simulink model "model"  (R2020a)
settings: Solver=FixedStepAuto  StartTime=0.0  StopTime=20  FixedStep=0.0001  RelTol=1e-3
values from neighbouring files (symbols this model uses):
  alp = Iz1 + (r1^2)*m1 + (l1^2)*m2 + (l1^2)*m3 + (l1^2)*m4    (= 1.69)    [Parameters.m]
  beta = Iz1 + Iz2 + Iz3 + Iz4 + (l2^2)*m3+ (l2^2)*m4 +m2*(r2^2)    (= 1.803225)    [Parameters.m]
  Ct_States1 = [Ct_States1;[x1, x2, x3, x4]]    [Parameters.m]
  Ct_timeS = [Ct_timeS;t]    [Parameters.m]
  d1 = 1.5    [Parameters.m]
  del = Iz3 + Iz4    (= 0.0201)    [Parameters.m]
  g = 9.81    [Parameters.m]
  gam = l1*l2*m3 + l1*l2*m4 + l1*m2*r2    (= 1.15)    [Parameters.m]
  k1 = 600    [Parameters.m]
  k2 = 100    [Parameters.m]
  l1 = 0.2    [Parameters.m]
  l2 = 0.25    [Parameters.m]
  m4 = 0.5    [Parameters.m]
  q0 = [0;0;0;0]    [Parameters.m]
settings Model: Creator=sirius  LastModifiedBy=sirius

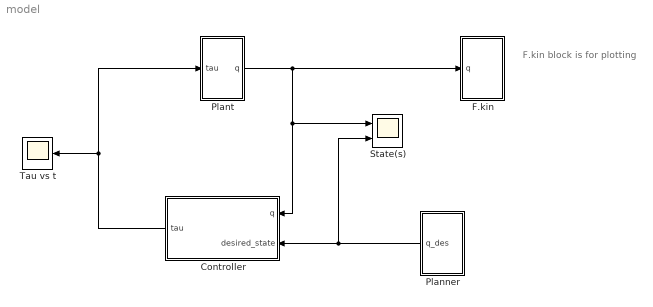
== system model ==
  note: F.kin block is for plotting
  Controller : Subsystem
  F.kin : Subsystem
  Planner : Subsystem
  Plant : Subsystem
  State(s) : Scope  NumInputPorts=2
  Tau vs t : Scope
  wires:
  Controller/1(tau) -> Tau vs t/1, Plant/1(tau)
  Planner/1(q_des) -> State(s)/2, Controller/2(desired_state)
  Plant/1(q) -> Controller/1(q), State(s)/1, F.kin/1(q)

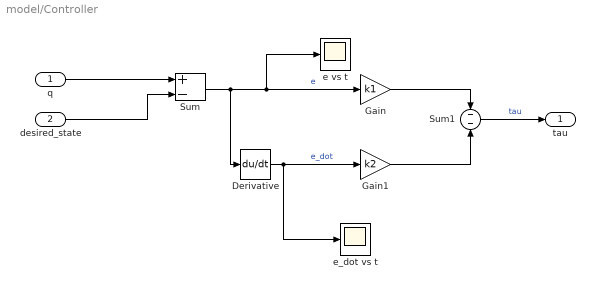
== system model/Controller ==
  q : Inport
  desired_state : Inport  Port=2
  Derivative : Derivative
  Gain : Gain  Gain=k1
  Gain1 : Gain  Gain=k2
  Sum : Sum  Inputs=+-
  Sum1 : Sum  Inputs=-|-
  e vs t : Scope
  e_dot vs t : Scope
  tau : Outport
  wires:
  q/1 -> Sum/1
  Gain/1 -> Sum1/1
  desired_state/1 -> Sum/2
  Derivative/1 -> e_dot vs t/1, Gain1/1  "e_dot"
  Sum1/1 -> tau/1  "tau"
  Gain1/1 -> Sum1/2
  Sum/1 -> e vs t/1, Gain/1, Derivative/1  "e"

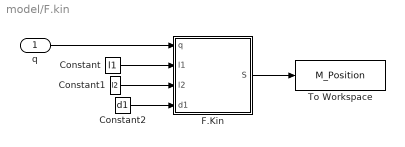
== system model/F.kin ==
  q : Inport
  Constant : Constant  Value=l1
  Constant1 : Constant  Value=l2
  Constant2 : Constant  Value=d1
  F.Kin : MATLAB Function  TreatAsAtomicUnit=on
  To Workspace : ToWorkspace  VariableName=M_Position  SampleTime=-1
  wires:
  Constant/1 -> F.Kin/2(l1)
  F.Kin/1(S) -> To Workspace/1
  Constant2/1 -> F.Kin/4(d1)
  q/1 -> F.Kin/1(q)
  Constant1/1 -> F.Kin/3(l2)

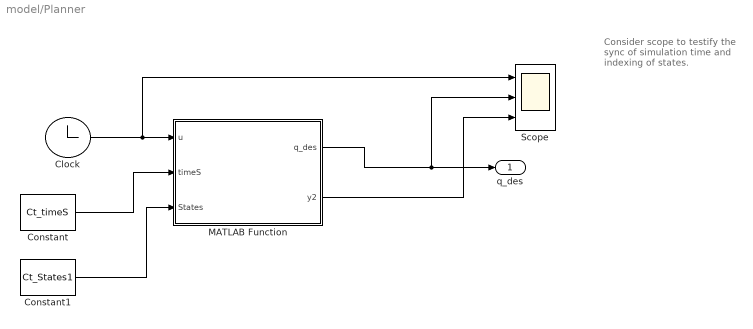
== system model/Planner ==
  note: Consider scope to testify the sync of simulation time and indexing of states.
  Clock : Clock
  Constant : Constant  Value=Ct_timeS
  Constant1 : Constant  Value=Ct_States1
  MATLAB Function : MATLAB Function  TreatAsAtomicUnit=on
  Scope : Scope  NumInputPorts=3
  q_des : Outport
  wires:
  MATLAB Function/2(y2) -> Scope/3
  Constant1/1 -> MATLAB Function/3(States)
  Clock/1 -> Scope/1, MATLAB Function/1(u)
  Constant/1 -> MATLAB Function/2(timeS)
  MATLAB Function/1(q_des) -> Scope/2, q_des/1

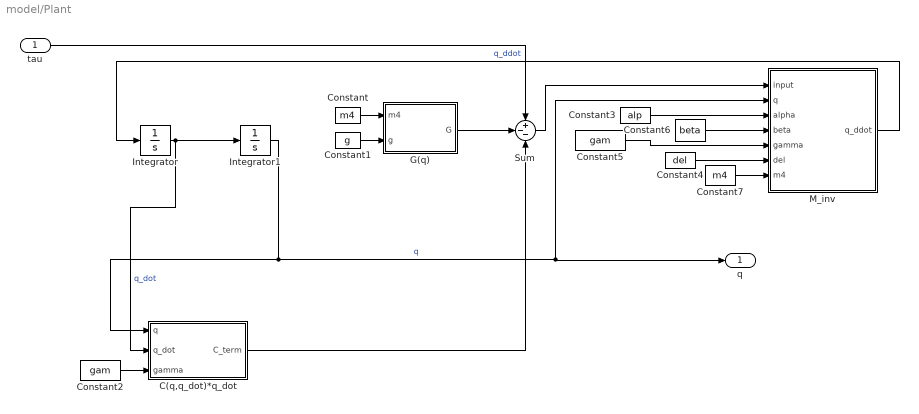
== system model/Plant ==
  tau : Inport
  C(q,q_dot)*q_dot : MATLAB Function  TreatAsAtomicUnit=on
  Constant : Constant  Value=m4
  Constant1 : Constant  Value=g
  Constant2 : Constant  Value=gam
  Constant3 : Constant  Value=alp
  Constant4 : Constant  Value=del
  Constant5 : Constant  Value=gam
  Constant6 : Constant  Value=beta
  Constant7 : Constant  Value=m4
  G(q) : MATLAB Function  TreatAsAtomicUnit=on
  Integrator : Integrator  InitialCondition=q0
  Integrator1 : Integrator  InitialCondition=q0
  M_inv : MATLAB Function  TreatAsAtomicUnit=on
  Sum : Sum  Inputs=+--
  q : Outport
  wires:
  M_inv/1(q_ddot) -> Integrator/1  "q_ddot"
  G(q)/1(G) -> Sum/2
  Integrator1/1 -> M_inv/2(q), q/1, C(q,q_dot)*q_dot/1(q)  "q"
  Integrator/1 -> Integrator1/1, C(q,q_dot)*q_dot/2(q_dot)  "q_dot"
  C(q,q_dot)*q_dot/1(C_term) -> Sum/3
  Sum/1 -> M_inv/1(input)
  Constant1/1 -> G(q)/2(g)
  Constant/1 -> G(q)/1(m4)
  Constant2/1 -> C(q,q_dot)*q_dot/3(gamma)
  Constant3/1 -> M_inv/3(alpha)
  Constant6/1 -> M_inv/4(beta)
  Constant5/1 -> M_inv/5(gamma)
  Constant4/1 -> M_inv/6(del)
  Constant7/1 -> M_inv/7(m4)
  tau/1 -> Sum/1

== matlab function model/Plant/G(q) ==
  data: m4 input; G output; g input
function G = gravity(m4,g)
G = [0;
     0;
     0;
     m4*g;
     ];

== matlab function model/Planner/MATLAB Function ==
  data: u input; q_des output; timeS input; States input; y2 output
function [q_des,y2] = fcn(u,timeS,States)
ind = (1 + round(u*100));
q_des = States(ind,:)';
y2 = timeS(ind);

== matlab function model/Plant/C(q,q_dot)*q_dot ==
  data: q input; C_term output; q_dot input; gamma input
function C_term = coriolis(q,q_dot,gamma)
C  = [-gamma*sin(q(2))*q_dot(2), -gamma*sin(q(2))*(q_dot(1)+q_dot(2)), 0, 0;
      -gamma*sin(q(2))*q_dot(1), 0, 0, 0; 
      0 , 0 , 0 , 0;
      0 , 0 , 0 , 0;] ; 
C_term  = C*q_dot;
end

== matlab function model/Plant/M_inv ==
  data: input input; q input; q_ddot output; alpha input; beta input; gamma input; del input; m4 input
function q_ddot = M_inverse(input,q, alpha , beta , gamma, del,m4)
M = [alpha + beta + 2*gamma*cos(q(2)) , beta + gamma*cos(q(2)), del, 0 ; 
     beta  + gamma*cos(q(2)), beta, del, 0;
     del, del, del,  0; 
     0, 0, 0, m4;];
q_ddot = M\input;

== matlab function model/F.kin/F.Kin ==
  data: q input; S output; l1 input; l2 input; d1 input
function S = fcn(q,l1,l2,d1)
S = [l1*cos(q(1)) + l2*cos(q(1)+q(2));
     l1*sin(q(1)) + l2*sin(q(1) + q(2));
     d1 - q(4);];
